simulink model "rocketSim"  (R2020b)
settings: Solver=VariableStepAuto  StartTime=0.0  StopTime=60  RelTol=1e-3
libraries: vrlib x3
settings Model: Creator=bean657  LastModifiedBy=Andreas

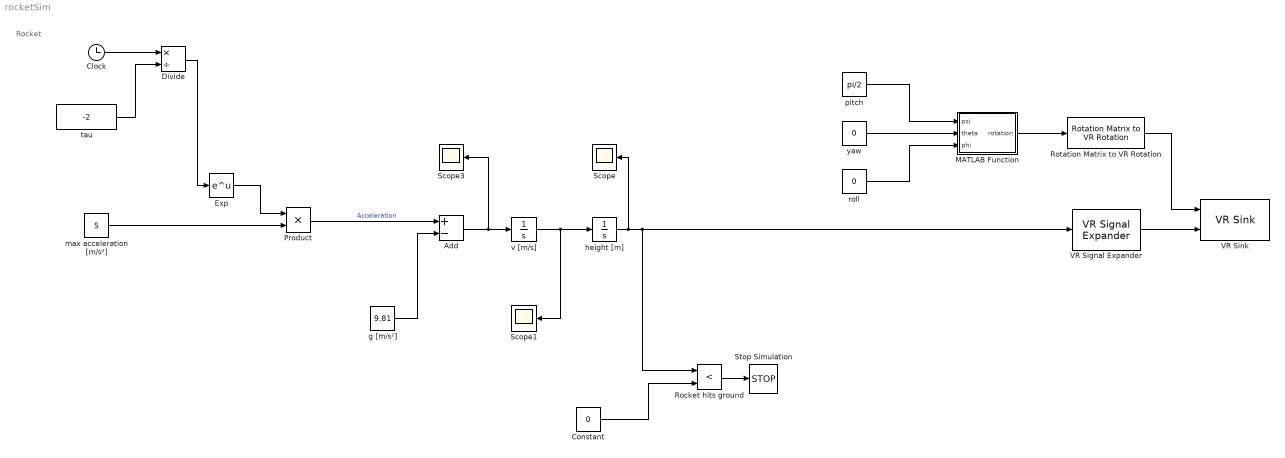
== system rocketSim ==
  note: Rocket
  Add : Sum  Inputs=+-
  Clock : Clock
  Constant : Constant  Value=0
  Divide : Product  Inputs=*/
  Exp : Math  SaturateOnIntegerOverflow=on
  MATLAB Function : MATLAB Function  TreatAsAtomicUnit=on
  Product : Product
  Rocket hits ground : RelationalOperator  Operator=<  OutDataTypeStr=boolean  RndMeth=Simplest
  Rotation Matrix to VR Rotation : vrlib/Utilities/Rotation Matrix to VR Rotation  maxzero=1e-12
      settings: SourceProductBaseCode=SL
  Scope : Scope
  Scope1 : Scope
  Scope3 : Scope
  Stop Simulation : Stop
  VR Signal Expander : vrlib/VR Signal Expander  outwidth=3  outidx=[2]
  VR Sink : vrlib/VR Sink  InstantiateOnLoad=on  SampleTime=0.1  ViewEnable=on  RemoteChange=off  RemoteView=off  FieldsWritten=Shuttle.rotation.4.1.1.double#Shuttle.translation.3.1.1.double  WorldFileName=rocketWorld.x3d  AutoView=off  VideoDimensions=[]  AllowVariableSize=off
  g [m/s²] : Constant  Value=9.81
  height [m] : Integrator
  max acceleration [m/s²] : Constant  Value=5
  pitch : Constant  Value=pi/2
  roll : Constant  Value=0
  tau : Constant  Value=-2
  v [m/s] : Integrator
  yaw : Constant  Value=0
  wires:
  max acceleration [m/s²]/1 -> Product/2
  Exp/1 -> Product/1
  Clock/1 -> Divide/1
  tau/1 -> Divide/2
  Divide/1 -> Exp/1
  Product/1 -> Add/1  "Acceleration"
  g [m/s²]/1 -> Add/2
  Add/1 -> Scope3/1, v [m/s]/1
  v [m/s]/1 -> Scope1/1, height [m]/1
  height [m]/1 -> Rocket hits ground/1, VR Signal Expander/1, Scope/1
  Rocket hits ground/1 -> Stop Simulation/1
  Constant/1 -> Rocket hits ground/2
  VR Signal Expander/1 -> VR Sink/2
  MATLAB Function/1(rotation) -> Rotation Matrix to VR Rotation/1
  pitch/1 -> MATLAB Function/1(psi)
  yaw/1 -> MATLAB Function/2(theta)
  roll/1 -> MATLAB Function/3(phi)
  Rotation Matrix to VR Rotation/1 -> VR Sink/1

== matlab function rocketSim/MATLAB Function ==
  data: psi input; rotation output; theta input; phi input
function rotation = fcn(psi,theta,phi)%yaw pitch roll

%yaw matrix
R3   = [ cos(psi) sin(psi) 0; 
             -sin(psi) cos(psi) 0; 
             0 0 1];
%pitch matrix
R2   = [cos(theta) 0 -sin(theta); 
        0  1           0; 
        sin(theta) 0  cos(theta)];
%roll matrix         
R1    = [1        0          0; 
         0  cos(phi)  sin(phi);
         0 -sin(phi)  cos(phi)];
         
         rotation = R1 * R2 * R3;
end
